simulink model "Ex_5"  (R2020a)
settings: Solver=VariableStepAuto  StartTime=0.0  StopTime=10  RelTol=1e-3
values from neighbouring files (symbols this model uses):
  B = 0.008    [m4.m]    (also in m5.m = 0)
  J = 0.093    [m4.m]    (also in m5.m = 1)
  La = 0.046    [m4.m]    (also in m5.m = 0.012)
  Laf = 1.8    [m5.m]
  Lf = 120    [m5.m]
  P = 2.5    [m5.m]
  Ra = 1    [m4.m]    (also in m5.m = 0.6)
  Rf = 240    [m5.m]
  Va = 220    [m4.m]    (also in m5.m = 240)
settings Model: Creator=abhin  LastModifiedBy=abhin

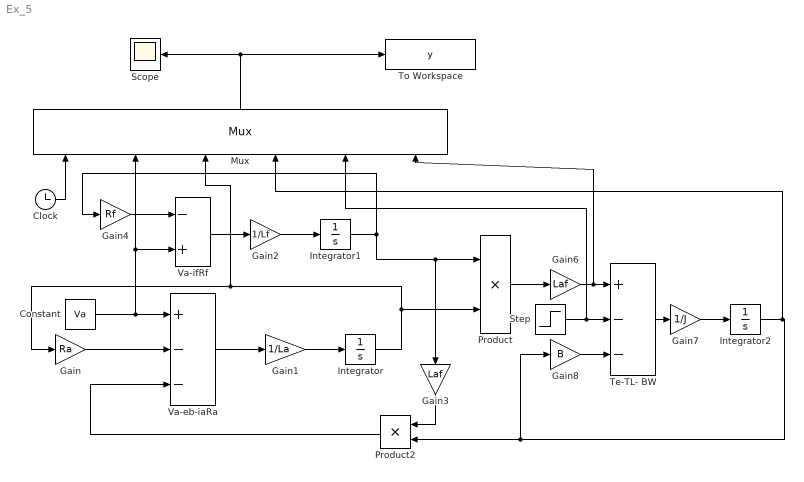
== system Ex_5 ==
  Clock : Clock
  Constant : Constant  Value=Va  SampleTime=1e-3
  Gain : Gain  Gain=Ra
  Gain1 : Gain  Gain=1/La
  Gain2 : Gain  Gain=1/Lf
  Gain3 : Gain  Gain=Laf
  Gain4 : Gain  Gain=Rf
  Gain6 : Gain  Gain=Laf
  Gain7 : Gain  Gain=1/J
  Gain8 : Gain  Gain=B
  Integrator : Integrator
  Integrator1 : Integrator
  Integrator2 : Integrator
  Mux : Mux  Inputs=6
  Product : Product
  Product2 : Product
  Scope : Scope
  Step : Step  Time=3  After=8*P  SampleTime=0
  Te-TL- BW : Sum  Inputs=+--
  To Workspace : ToWorkspace  VariableName=y  SaveFormat=Structure  SampleTime=-1
      settings: Save2DSignal=2-D array (concatenate along first dimension)
  Va-eb-iaRa : Sum  Inputs=+--
  Va-ifRf : Sum  Inputs=-+
  wires:
  Gain/1 -> Va-eb-iaRa/2
  Constant/1 -> Va-eb-iaRa/1, Va-ifRf/2, Mux/2
  Va-eb-iaRa/1 -> Gain1/1
  Gain1/1 -> Integrator/1
  Integrator/1 -> Product/2, Mux/3, Gain/1
  Va-ifRf/1 -> Gain2/1
  Gain2/1 -> Integrator1/1
  Integrator1/1 -> Gain4/1, Gain3/1, Product/1
  Product/1 -> Gain6/1
  Gain6/1 -> Mux/6, Te-TL- BW/1
  Te-TL- BW/1 -> Gain7/1
  Gain8/1 -> Te-TL- BW/3
  Gain3/1 -> Product2/1
  Product2/1 -> Va-eb-iaRa/3
  Clock/1 -> Mux/1
  Mux/1 -> To Workspace/1, Scope/1
  Step/1 -> Mux/5, Te-TL- BW/2
  Gain4/1 -> Va-ifRf/1
  Gain7/1 -> Integrator2/1
  Integrator2/1 -> Mux/4, Gain8/1, Product2/2
